simulink model "grace"  (Simulink 8.1)
settings: Solver=ode45  StartTime=0.0  StopTime=40  RelTol=1e-3
values from neighbouring files (symbols this model uses):
  Sample_time = 0.001    [script.m]
libraries: cstblocks x12, simulink x2
settings Model: Creator=PhM  LastModifiedBy=dello
settings DataIOCC: LimitDataPoints=off  SignalLoggingSaveFormat=Dataset
settings OptimizationCC: InitFltsAndDblsToZero=on
settings DebuggingCC: SaveWithParameterizedLinksMsg=none  SignalResolutionControl=TryResolveAllWithWarning  MultiTaskDSMMsg=warning  MultiTaskCondExecSysMsg=none  StrictBusMsg=None
settings RTWCC: IncludeERTFirstTime=on
settings GRTTargetCC: TargetFcnLib=ansi_tfl_tmw.mat

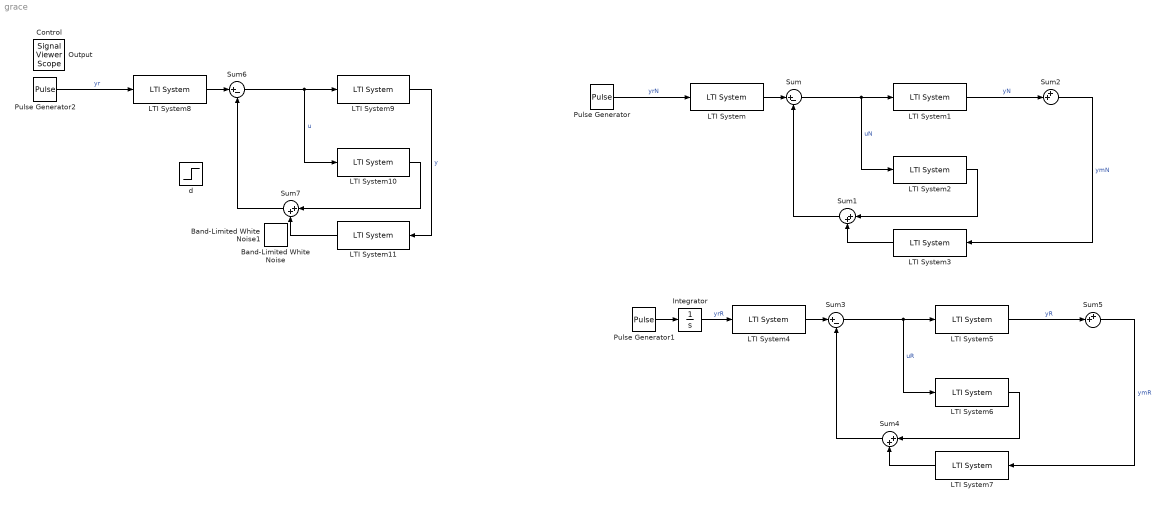
== system grace ==
  Integrator : Integrator
  LTI System : cstblocks/LTI System  sys=hs  IC=[]
  LTI System1 : cstblocks/LTI System  sys=Gs  IC=[]
  LTI System10 : cstblocks/LTI System  sys=Cus  IC=[]
  LTI System11 : cstblocks/LTI System  sys=Cys  IC=[]
  LTI System2 : cstblocks/LTI System  sys=Cus  IC=[]
  LTI System3 : cstblocks/LTI System  sys=Cys  IC=[]
  LTI System4 : cstblocks/LTI System  sys=hs  IC=[]
  LTI System5 : cstblocks/LTI System  sys=Gs  IC=[]
  LTI System6 : cstblocks/LTI System  sys=Cus  IC=[]
  LTI System7 : cstblocks/LTI System  sys=Cys  IC=[]
  LTI System8 : cstblocks/LTI System  sys=hs  IC=[]
  LTI System9 : cstblocks/LTI System  sys=Gs  IC=[]
  Pulse Generator : DiscretePulseGenerator  PulseType=Time based  Period=4  PulseWidth=50
  Pulse Generator1 : DiscretePulseGenerator  PulseType=Time based  Period=4  PulseWidth=50
  Pulse Generator2 : DiscretePulseGenerator  PulseType=Time based  Period=4  PulseWidth=50
  Sum : Sum  Inputs=|+-
  Sum1 : Sum  Inputs=|++
  Sum2 : Sum  Inputs=++|
  Sum3 : Sum  Inputs=|+-
  Sum4 : Sum  Inputs=|++
  Sum5 : Sum  Inputs=++|
  Sum6 : Sum  Inputs=|+-
  Sum7 : Sum  Inputs=|++
  Band-Limited White Noise : simulink/Sources/Band-Limited White Noise  IOType=siggen  Cov=Noise_ramp  Ts=Sample_time  seed=[23341]
  Band-Limited White Noise1 : simulink/Sources/Band-Limited White Noise  IOType=siggen  Cov=Noise_step  Ts=Sample_time  seed=[23341]
  Control : SignalViewerScope  IOType=viewer  NumInputPorts=2  RefreshTime=0.035000
      settings: YMin=-5~-5  YMax=5~5
  Output : SignalViewerScope  IOType=viewer  NumInputPorts=2  LegendLocations="0.92661     0.84402    0.051611    0.096574 0.92295     0.42219    0.053807    0.066509"  RefreshTime=0.035000
      settings: ShowLegends=on  TimeRange=40  YMin=-2~-2  YMax=2.25~2.25
  d : Step  IOType=siggen  Time=10  After=0  SampleTime=0.001
  wires:
  Pulse Generator/1 -> LTI System/1  "yrN"
  LTI System/1 -> Sum/1
  Sum/1 -> LTI System2/1, LTI System1/1  "uN"
  LTI System2/1 -> Sum1/1
  LTI System3/1 -> Sum1/2
  Sum1/1 -> Sum/2
  LTI System1/1 -> Sum2/2  "yN"
  Sum2/1 -> LTI System3/1  "ymN"
  Pulse Generator1/1 -> Integrator/1
  LTI System4/1 -> Sum3/1
  Sum3/1 -> LTI System6/1, LTI System5/1  "uR"
  LTI System6/1 -> Sum4/1
  LTI System7/1 -> Sum4/2
  Sum4/1 -> Sum3/2
  LTI System5/1 -> Sum5/2  "yR"
  Sum5/1 -> LTI System7/1  "ymR"
  Integrator/1 -> LTI System4/1  "yrR"
  Pulse Generator2/1 -> LTI System8/1  "yr"
  LTI System8/1 -> Sum6/1
  Sum6/1 -> LTI System10/1, LTI System9/1  "u"
  LTI System10/1 -> Sum7/1
  LTI System11/1 -> Sum7/2
  Sum7/1 -> Sum6/2
  LTI System9/1 -> LTI System11/1  "y"
